simulink model "SOC_Estimation_EKF"  (R2020b)
settings: Solver=FixedStepDiscrete  StartTime=0.0  StopTime=simtime  FixedStep=0.1  RelTol=1e-3
values from neighbouring files (symbols this model uses):
  cell_model = ekfData.model    [iterEKF.m]
  dt = deltat    [cell_model_loadfile_SOCEst.m]
  ekfData = initializeEKF_3NP(voltage(1),T,SigmaX0,SigmaV,SigmaW,cell_model,numpoles)    [SSG_EKF_Estimation.m]    (also in cell_model_loadfile_SOCEst.m)
  numpoles = 2    [SSG_EKF_Estimation.m]    (also in cell_model_loadfile_SOCEst.m)
  R0 = zeros(numpoles,1)    [cell_model_loadfile_SOCEst.m]    (also in iterEKF.m = getParamESC('R0Param',Tk,cell_model); iterationEKF.m = getParamESC('R0Param',Tk,model); iterationEKF_3NP.m = getParamESC('R0Param',Tk,model))
  simtime = length(DYNData.script1.current)*0.1    [cell_model_loadfile_SOCEst.m]
  T = 25    [SSG_EKF_Estimation.m]    (also in cell_model_loadfile_SOCEst.m = 40)
undefined symbols (not defined in the file or in its folder): DYNData
libraries: simulink x2
settings Model: Creator=Lenovo  LastModifiedBy=Lenovo
settings DataIOCC: ReturnWorkspaceOutputs=off

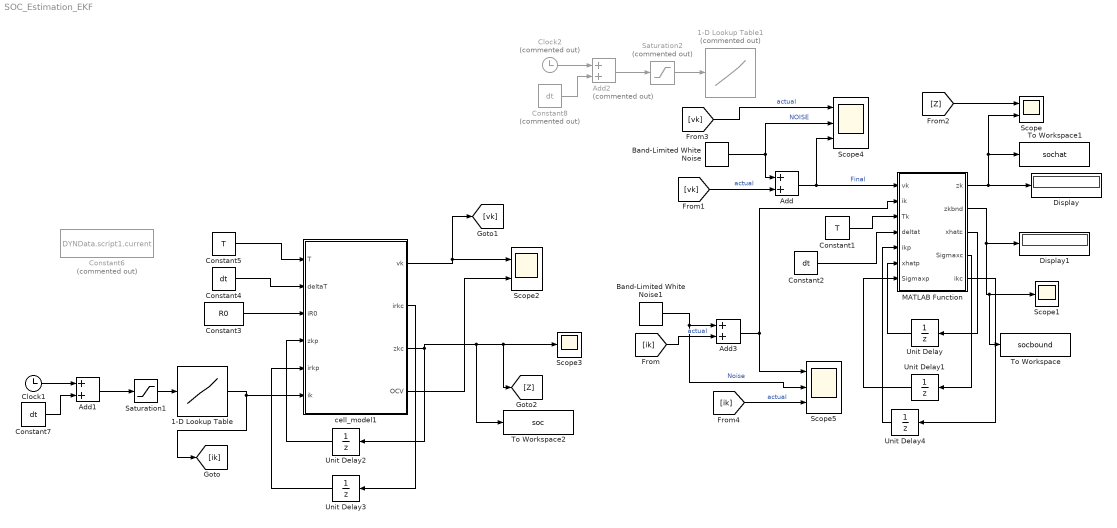
== system SOC_Estimation_EKF ==
  1-D Lookup Table : Lookup_n-D  NumberOfTableDimensions=1  LookupTableObject=''  BreakpointsForDimension1=0.1*(1:length(DYNData.script1.current))  BreakpointsForDimension1FirstPoint=10  BreakpointsForDimension2FirstPoint=10  BreakpointsForDimension1Spacing=12  BreakpointsForDimension2Spacing=12  IndexSearchMethod=Evenly spaced points  Table=DYNData.script1.current  InterpMethod=Nearest  DiagnosticForOutOfRangeInput=Error  InternalRulePriority=Speed  RndMeth=Simplest  InputSameDT=on
  1-D Lookup Table1 : Lookup_n-D  Commented=on  NumberOfTableDimensions=1  LookupTableObject=''  BreakpointsForDimension1=0.1*(1:length(DYNData.script1.voltage))  BreakpointsForDimension1FirstPoint=10  BreakpointsForDimension2FirstPoint=10  BreakpointsForDimension1Spacing=12  BreakpointsForDimension2Spacing=12  IndexSearchMethod=Evenly spaced points  Table=DYNData.script1.voltage  InterpMethod=Nearest  DiagnosticForOutOfRangeInput=Error  InternalRulePriority=Speed  RndMeth=Simplest  InputSameDT=on
  Add : Sum
  Add1 : Sum
  Add2 : Sum  Commented=on
  Add3 : Sum
  Band-Limited White Noise : simulink/Sources/Band-Limited White Noise  Cov=[0.01]  Ts=0.1  seed=[23341]
  Band-Limited White Noise1 : simulink/Sources/Band-Limited White Noise  Cov=[0.1]  Ts=0.1  seed=[23341]
  Clock1 : Clock
  Clock2 : Clock  Commented=on
  Constant1 : Constant  Value=T
  Constant2 : Constant  Value=dt
  Constant3 : Constant  Value=R0
  Constant4 : Constant  Value=dt
  Constant5 : Constant  Value=T
  Constant6 : Constant  Commented=on  Value=DYNData.script1.current
  Constant7 : Constant  Value=dt
  Constant8 : Constant  Commented=on  Value=dt
  Display : Display
  Display1 : Display
  MATLAB Function : MATLAB Function  TreatAsAtomicUnit=on
  Saturation1 : Saturate  UpperLimit=simtime
  Saturation2 : Saturate  Commented=on  UpperLimit=simtime
  Scope : Scope  NumInputPorts=2
  Scope1 : Scope
  Scope2 : Scope  NumInputPorts=2
  Scope3 : Scope
  Scope4 : Scope  NumInputPorts=3
  Scope5 : Scope  NumInputPorts=3
  To Workspace : ToWorkspace  VariableName=socbound  SampleTime=-1
  To Workspace1 : ToWorkspace  VariableName=sochat  SampleTime=-1
  To Workspace2 : ToWorkspace  VariableName=soc  SampleTime=-1
  Unit Delay : UnitDelay  InitialCondition=ekfData.xhat  SampleTime=-1  HasFrameUpgradeWarning=on
  Unit Delay1 : UnitDelay  InitialCondition=ekfData.SigmaX  SampleTime=-1  HasFrameUpgradeWarning=on
  Unit Delay2 : UnitDelay  InitialCondition=1  SampleTime=-1  HasFrameUpgradeWarning=on
  Unit Delay3 : UnitDelay  SampleTime=-1  HasFrameUpgradeWarning=on
  Unit Delay4 : UnitDelay  InitialCondition=ekfData.priorI  SampleTime=-1  HasFrameUpgradeWarning=on
  cell_model1 : MATLAB Function  TreatAsAtomicUnit=on
  wires:
  Unit Delay3/1 -> cell_model1/5(irkp)
  Constant5/1 -> cell_model1/1(T)
  Constant3/1 -> cell_model1/3(iR0)
  cell_model1/2(irkc) -> Unit Delay3/1
  cell_model1/3(zkc) -> To Workspace2/1, [Z], Scope3/1, Unit Delay2/1
  Constant4/1 -> cell_model1/2(deltaT)
  Unit Delay2/1 -> cell_model1/4(zkp)
  1-D Lookup Table/1 -> [ik], cell_model1/6(ik)
  Clock1/1 -> Add1/1
  Constant7/1 -> Add1/2
  Add1/1 -> Saturation1/1
  Saturation1/1 -> 1-D Lookup Table/1
  cell_model1/4(OCV) -> Scope2/2
  cell_model1/1(vk) -> [vk], Scope2/1
  Constant1/1 -> MATLAB Function/3(Tk)
  Constant2/1 -> MATLAB Function/4(deltat)
  MATLAB Function/1(zk) -> To Workspace1/1, Scope/2, Display/1
  MATLAB Function/2(zkbnd) -> To Workspace/1, Scope1/1, Display1/1
  [Z] -> Scope/1
  MATLAB Function/3(xhatc) -> Unit Delay/1
  MATLAB Function/4(Sigmaxc) -> Unit Delay1/1
  MATLAB Function/5(ikc) -> Unit Delay4/1
  Unit Delay/1 -> MATLAB Function/6(xhatp)
  Unit Delay1/1 -> MATLAB Function/7(Sigmaxp)
  Unit Delay4/1 -> MATLAB Function/5(ikp)
  Saturation2/1 -> 1-D Lookup Table1/1
  Add2/1 -> Saturation2/1
  Constant8/1 -> Add2/2
  Clock2/1 -> Add2/1
  Band-Limited White Noise/1 -> Scope4/2, Add/1  "NOISE"
  [vk] -> Add/2  "actual"
  Band-Limited White Noise1/1 -> Scope5/2, Add3/1  "Noise"
  [ik] -> Add3/2  "actual"
  Add/1 -> MATLAB Function/1(vk), Scope4/3  "Final"
  Add3/1 -> MATLAB Function/2(ik), Scope5/1
  [vk] -> Scope4/1  "actual"
  [ik] -> Scope5/3  "actual"

== matlab function SOC_Estimation_EKF/MATLAB Function ==
  data: vk input size=1; zk output size=1; ik input size=1; Tk input; deltat input; zkbnd output size=1; ekfData parameter; numpoles parameter; xhatc output; Sigmaxc output; ikc output; ikp input; xhatp input; Sigmaxp input; cell_model parameter
function [zk,zkbnd,xhatc,Sigmaxc,ikc] = fcn(vk,ik,Tk,deltat,ekfData,numpoles,ikp,xhatp,Sigmaxp,cell_model) 
  
  
  % Load the cell model parameters
  Q  = getParamESC('QParam',Tk,cell_model);
  G  = getParamESC('GParam',Tk,cell_model);
  M  = getParamESC('MParam',Tk,cell_model);
  M0 = getParamESC('M0Param',Tk,cell_model);
  RC = exp(-deltat./abs(getParamESC('RCParam',Tk,cell_model)))';
  R  = getParamESC('RParam',Tk,cell_model)';
  R0 = getParamESC('R0Param',Tk,cell_model);
  eta = getParamESC('etaParam',Tk,cell_model);
%   if ik<0, ik=ik*eta; end
  
% ik(ik<0) = eta.*ik(ik<0);
 ik = ik(:);
 etaik = ik; 
  for iii=1:length(ik)
    if etaik(iii)<0
        etaik(iii) = eta*ik(iii); % compensate for coulombic efficiency
    end
    ik(iii)=etaik(iii);
  end
  
  % Get data stored in ekfData structure
%   I = ekfData.priorI;
%   xhat = ekfData.xhat;
%   SigmaX = ekfData.SigmaX;
  I=ikp;
  xhat=xhatp;
  SigmaX=Sigmaxp;
  SigmaV = ekfData.SigmaV;
  SigmaW = ekfData.SigmaW;
  
% irInd = ekfData.irInd;
  irInd1 = ekfData.irInd1;
% irInd2 = ekfData.irInd2;
% irInd3 = ekfData.irInd3;
  hkInd = ekfData.hkInd;
  zkInd = ekfData.zkInd;
%   if abs(ik)>Q/100, ekfData.signIk = sign(ik); end
  signIk = ekfData.signIk;
  %ekfdata.signIk(abs(ik)>Q/100) = sign(ik);
  
  % EKF Step 0: Compute Ahat[k-1], Bhat[k-1]
  nx = length(xhat); Ahat = zeros(nx,nx); Bhat = zeros(nx,1);
  Ahat(zkInd,zkInd) = 1; Bhat(zkInd) = -deltat/(3600*Q);
% Ahat(irInd,irInd) = diag(RC); Bhat(irInd) = 1-RC(:);
  for ii=1:numpoles
      Ahat(ii,ii) = RC(ii); Bhat(ii) = 1-RC(ii);
%     Ahat(irInd1,irInd1) = diag(RC); Bhat(irInd1) = 1-RC(:);
  end
% Ahat(irInd2,irInd2) = diag(RC); Bhat(irInd2) = 1-RC(:);
% Ahat(irInd3,irInd3) = diag(RC); Bhat(irInd2) = 1-RC(:);
% Ahat(irInd3,irInd3) = diag(RC); Bhat(irInd3) = 1-RC(:);
  Ah  = exp(-abs(I*G*deltat/(3600*Q)));  % hysteresis factor
  Ahat(hkInd,hkInd) = Ah;
  B = [Bhat, 0*Bhat];
  Bhat(hkInd) = -abs(G*deltat/(3600*Q))*Ah*(1+sign(I)*xhat(hkInd));
  B(hkInd,2) = Ah-1;
  
  % Step 1a: State estimate time update
  xhat = Ahat*xhat + B*[I; sign(I)]; 
  xhat(hkInd) = min(1,max(-1,xhat(hkInd)));
  xhat(zkInd) = min(1.05,max(-0.05,xhat(zkInd)));

  % Step 1b: Error covariance time update
  %          sigmaminus(k) = Ahat(k-1)*sigmaplus(k-1)*Ahat(k-1)' + ...
  %                          Bhat(k-1)*sigmawtilde*Bhat(k-1)'
%   SigmaX = Ahat*SigmaX*Ahat' + Bhat*SigmaW*Bhat';
    SigmaX = Ahat*SigmaX*Ahat' + Bhat*SigmaW*Bhat';
  
  % Step 1c: Output estimate
  yhat = OCVfromSOCtemp(xhat(zkInd),Tk,cell_model) + M0*signIk + ...
         M*xhat(hkInd) - R'*xhat(irInd1) - R0*ik;
%          OCVfromSOCtemp(xhat(zkInd),Tk,model) + M0*signIk + ...
%          M*xhat(hkInd) - R.*xhat(irInd1) - R.*xhat(irInd2) - R.*xhat(irInd3) - R0*ik];
%   yhat(6,:) = [];
  
  % Step 2a: Estimator gain matrix
  Chat = zeros(1,nx);
  Chat(zkInd) = dOCVfromSOCtemp(xhat(zkInd),Tk,cell_model);
  Chat(hkInd) = M;
  Chat(irInd1) = -R;
%   Chat(irInd2) = -R;
%   Chat(irInd3) = -R;
  Dhat = 1;
  SigmaY = Chat*SigmaX*Chat' + Dhat*SigmaV*Dhat';
  L = SigmaX*Chat'/SigmaY;
  
  % Step 2b: State estimate measurement update
  r = vk - yhat; % residual.  Use to check for sensor errors...
  if r^2 > 100*SigmaY, L(:)=0.0; end 
  xhat = xhat + L*r;
  xhat(hkInd) = min(1,max(-1,xhat(hkInd))); % Help maintain robustness
  xhat(zkInd) = min(1.05,max(-0.05,xhat(zkInd)));
  
  % Step 2c: Error covariance measurement update
  SigmaX = SigmaX - L*SigmaY*L';
  %   % Q-bump code
  if r^2 > 4*SigmaY % bad voltage estimate by 2 std. devs, bump Q 
    fprintf('Bumping SigmaX\n');
    SigmaX(zkInd,zkInd) = SigmaX(zkInd,zkInd)*ekfData.Qbump;
  end
  [~,S,V] = svd(SigmaX);
  HH = V*S*V';
  SigmaX = (SigmaX + SigmaX' + HH + HH')/4; % Help maintain robustness
  
  % Save data in ekfData structure for next time...
  ikc = ik;
  Sigmaxc = SigmaX;
  xhatc = xhat;
%     ekfData.priorI = ik;
%   ekfData.SigmaX = SigmaX;
%   ekfData.xhat = xhat;
  zk = xhat(zkInd);
  zkbnd = 3*sqrt(SigmaX(zkInd,zkInd));
  
%getparamESC  
function theParam = getParamESC(paramName,temp,model)
%   theFields = fields(model); % get list of fields stored in model
%   match = strcmpi(paramName,theFields); % see if any match desired data
%   if ~match, % if not, throw an error
%     error('Parameter "%s" does not exist in model',paramName);
%   end
  fieldName = char(paramName); % case-sensitive field name

  % if model contains data at only one temperature
  if isscalar(model.temps)
    if model.temps ~= temp % check whether requested data exists
      error('Model does not contain requested data at this temperature');
    end
    theParam = model.(fieldName);
    return
  end

  % Otherwise, model has multiple temperatures. Bound input "temp" between
  % mininum and maximum stored temperature to prohibit "NaN" in output
  theParamData = model.(fieldName);
  temp = max(min(temp,max(model.temps)),min(model.temps)); 
  ind = find(model.temps == temp); % see if there is an exact match to
  if ~isempty(ind), % avoid call to (slow) interp1 whenever possible
    if size(theParamData,1) == 1,
      theParam = theParamData(ind);
    else
      theParam = theParamData(ind,:);
    end
  else % if there is not an exact match, we interpolate between parameter
    theParam = interp1(model.temps,theParamData,temp,'spline'); % values
  end  % stored at different temperatures
end
end

== matlab function SOC_Estimation_EKF/cell_model1 ==
  data: vk output size=1; irkc output size=numpoles; T input; deltaT input; iR0 input; zkp input; irkp input; cell_model parameter; ik input; zkc output size=1; OCV output size=1

% function [vk,irk,hk,zk,sik,OCV] = simCell(ik,T,deltaT,model,z0,iR0,h0)
% 
% Simulates an ESC model for input current ik at temperature T
%
% Inputs:  ik - current, where (+) is discharge
%          T  - temperature (degC)
%      deltaT - sampling interval in data (s)
%       model - standard model structure
%          z0 - initial cell state of charge
%         iR0 - initial resistor currents as column vector
%          h0 - initial hysteresis state
% Outputs: vk - cell voltage for all timesteps
%         irk - resistor currents (in R-C branches) for all timesteps
%          hk - hysteresis states for all timesteps
%          zk - state of charge for all timesteps
%         sik - instantaneous hysteresis for all timesteps
%         OCV - open-circuit voltage for all timesteps

% Copyright (c) 2015 by Gregory L. Plett of the University of Colorado 
% Colorado Springs (UCCS). This work is licensed under a Creative Commons 
% Attribution-NonCommercial-ShareAlike 4.0 Intl. License, v. 1.0.
% It is provided "as is", without express or implied warranty, for 
% educational and informational purposes only.
%
% This file is provided as a supplement to: Plett, Gregory L., "Battery
% Management Systems, Volume I, Battery Modeling," Artech House, 2015.

function [vk,irkc,zkc,OCV] = cellmodel(T,deltaT,iR0,zkp,irkp, cell_model,ik)
  % Force data to be column vector(s)
  
%   ik=[DYNData.script1.current(round(t*10)),DYNData.script1.current(round(t*10)+1)];
  %vact=interp1(0.1*(1:length(DYNData.script1.voltage)),DYNData.script1.voltage,t,'nearest');
  %ik=interp1(0.1*(1:length(DYNData.script1.current)),DYNData.script1.current,t,'nearest');
  ik = ik(:); iR0 = iR0(:);
%   vk=zeros(1,1); zkc=zeros(1,1); OCV=zeros(1,1); irkc=zeros(numpoles,1);
 %Get model parameters from model structure
  RCfact = exp(-deltaT./abs(getParamESC('RCParam',T,cell_model)))';
 %G = getParamESC('GParam',T,model);
  Q = getParamESC('QParam',T,cell_model);
 %M = getParamESC('MParam',T,model);
 %M0 = getParamESC('M0Param',T,model);
  RParam = getParamESC('RParam',T,cell_model);
  R0Param = getParamESC('R0Param',T,cell_model);
  etaParam = getParamESC('etaParam',T,cell_model);
  
  etaik = ik; 
  for iii=1:length(ik)
    if etaik(iii)<0
        etaik(iii) = etaParam*ik(iii); % compensate for coulombic efficiency
    end
  end
  % Simulate the dynamic states of the model

    irkc = RCfact.*irkp + (1-RCfact)*etaik;
    zkc = zkp-etaik*deltaT/(Q*3600); 
    
  % Compute output equation
  OCV = OCVfromSOCtemp(zkc,T,cell_model);
  vk = OCV - RParam*irkc - ik.*R0Param ;%+ M*hk + M0*sik;

  %verr=vact-vk;


function theParam = getParamESC(paramName,temp,model)
%   theFields = fields(model); % get list of fields stored in model
%   match = strcmpi(paramName,theFields); % see if any match desired data
%   if ~match, % if not, throw an error
%     error('Parameter "%s" does not exist in model',paramName);
%   end
%   fieldName = char(theFields(match)); % case-sensitive field name

  % if model contains data at only one temperature
  if isscalar(model.temps),
    if model.temps ~= temp, % check whether requested data exists
      error('Model does not contain requested data at this temperature');
    end
    theParam = model.(paramName);
    return
  end

  % Otherwise, model has multiple temperatures. Bound input "temp" between
  % mininum and maximum stored temperature to prohibit "NaN" in output
  theParamData = model.(paramName);
  temp = max(min(temp,max(model.temps)),min(model.temps)); 
  ind = find(model.temps == temp); % see if there is an exact match to
  if ~isempty(ind), % avoid call to (slow) interp1 whenever possible
    if size(theParamData,1) == 1,
      theParam = theParamData(ind);
    else
      theParam = theParamData(ind,:);
    end
  else % if there is not an exact match, we interpolate between parameter
    theParam = interp1(model.temps,theParamData,temp,'spline'); % values
  end  % stored at different temperatures
  
% function ocv = OCVfromSOCtemp(soc,temp,model)
%
% Computes the fully rested open-circuit voltage for a particular state of 
% charge and temperature point
%
% Inputs: soc = scalar or matrix of cell state of charge points
%        temp = scalar or matrix of temperatures at which to calc. OCV
%       model = data structure produced by processDynamic
% Output: ocv = scalar or matrix of open circuit voltages -- one for every
%               soc and temperature input point

% Copyright (c) 2015 by Gregory L. Plett of the University of Colorado 
% Colorado Springs (UCCS). This work is licensed under a Creative Commons 
% Attribution-NonCommercial-ShareAlike 4.0 Intl. License, v. 1.0.
% It is provided "as is", without express or implied warranty, for 
% educational and informational purposes only.
%
% This file is provided as a supplement to: Plett, Gregory L., "Battery
% Management Systems, Volume I, Battery Modeling," Artech House, 2015.

function ocv=OCVfromSOCtemp(soc,temp,model)
  soccol = soc(:); % force soc to be column vector
  SOC = model.SOC(:); % force to be column vector
  OCV0 = model.OCV0(:); % force to be column vector
  OCVrel = model.OCVrel(:); % force to be column vector
  if isscalar(temp), % replicate a scalar temperature for all socs
    tempcol = temp*ones(size(soccol)); 
  else
    tempcol = temp(:); % force matrix temperature to be column vector
    if ~isequal(size(tempcol),size(soccol)),
      error(['Function inputs "soc" and "temp" must either have same '...
        'number of elements, or "temp" must be a scalar']);
    end
  end
  diffSOC=SOC(2)-SOC(1); % spacing between SOC points - assume uniform
  ocv=zeros(size(soccol)); % initialize output to zero
  I1=find(soccol <= SOC(1)); % indices of socs below model-stored data
  I2=find(soccol >= SOC(end)); % and of socs above model-stored data
  I3=find(soccol > SOC(1) & soccol < SOC(end)); % the rest of them
  I6=isnan(soccol); % if input is "not a number" for any locations

  % for voltages less than lowest stored soc datapoint, extrapolate off 
  % low end of table 
  if ~isempty(I1),
    dv = (OCV0(2)+tempcol.*OCVrel(2)) - (OCV0(1)+tempcol.*OCVrel(1));
    ocv(I1)= (soccol(I1)-SOC(1)).*dv(I1)/diffSOC + ...
             OCV0(1)+tempcol(I1).*OCVrel(1);
  end

  % for voltages greater than highest stored soc datapoint, extrapolate off
  % high end of table
  if ~isempty(I2),
    dv = (OCV0(end)+tempcol.*OCVrel(end)) - ...
         (OCV0(end-1)+tempcol.*OCVrel(end-1));
    ocv(I2) = (soccol(I2)-SOC(end)).*dv(I2)/diffSOC + ...
              OCV0(end)+tempcol(I2).*OCVrel(end);
  end

  % for normal soc range, manually interpolate (10x faster than "interp1")
  I4=(soccol(I3)-SOC(1))/diffSOC; % using linear interpolation
  I5=floor(I4); I45 = I4-I5; omI45 = 1-I45;
  ocv(I3)=OCV0(I5+1).*omI45 + OCV0(I5+2).*I45;
  ocv(I3)=ocv(I3) + tempcol(I3).*(OCVrel(I5+1).*omI45 + OCVrel(I5+2).*I45);
  ocv(I6)=0; % replace NaN SOCs with zero voltage
  ocv = reshape(ocv,size(soc)); % output is same shape as input
